simulink library "FG_Controller_Library"  (R2017b)
settings: Solver=VariableStepAuto  StartTime=0.0  StopTime=10.0  RelTol=1e-3
undefined symbols (not defined in the file or in its folder): fcut_velocity_joint, GaitLibrary, isSim, UserParams
libraries: slrtlib x113, simulink x1, func_block_library x1
(part 1 of 3)
settings Model: Creator=81068  LastModifiedBy=hanli

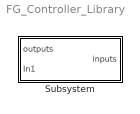
== system FG_Controller_Library ==
  Subsystem : Subsystem

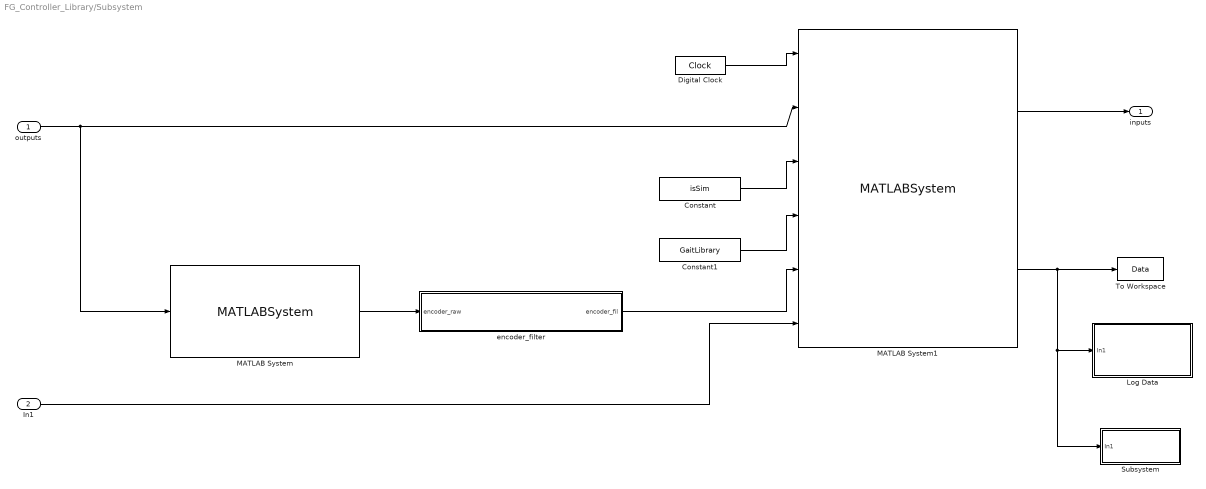
== system FG_Controller_Library/Subsystem ==
  outputs : Inport  OutDataTypeStr=Bus: CassieOutBus
  In1 : Inport  Port=2
  Constant : Constant  Value=isSim  OutDataTypeStr=boolean  LockScale=on
  Constant1 : Constant  Value=GaitLibrary  OutDataTypeStr=Bus: cassieGaitLibraryBus  LockScale=on
  Digital Clock : DigitalClock  SampleTime=UserParams.SampleTime
  Log Data : Subsystem
  MATLAB System : MATLABSystem  System=ExtractJointPosition  SimulateUsing=Code generation
      mask Type: ExtractJointPosition
      mask Display:
      | disp('ExtractJointPosition');
      | port_label('input',1,'cassieOutputs');
      | port_label('output',1,'JointPosition');
  MATLAB System1 : MATLABSystem  System=FG_Controller  Kp_pitch=c_Kp_pitch  Kd_pitch=c_Kd_pitch  Kp_roll=c_Kp_roll  Kd_roll=c_Kd_roll  Kp_yaw=c_Kp_yaw  Kd_yaw=c_Kd_yaw  Kp_abduction=c_Kp_abduction  Kp_rotation=c_Kp_rotation  Kp_thigh=c_Kp_thigh  Kp_knee=c_Kp_knee  Kp_toe=c_Kp_toe  Kd_abduction=c_Kd_abduction  Kd_rotation=c_Kd_rotation  Kd_thigh=c_Kd_thigh  Kd_knee=c_Kd_knee  Kd_toe=c_Kd_toe  Kfs_p=c_Kfs_p  Kfl_p=c_Kfl_p  Kfs_d=c_Kfs_d  Kfl_d=c_Kfl_d  Kp_toe_stand=c_Kp_toe_stand  Kd_toe_stand=c_Kd_toe_stand  Kp_lateral_stand=c_Kp_lateral_stand  Kd_lateral_stand=c_Kd_lateral_stand  Kp_abduction_stand=c_Kp_abduction_stand  Kd_abduction_stand=c_Kd_abduction_stand  Kp_thigh_stand=c_Kp_thigh_stand  Kd_thigh_stand=c_Kd_thigh_stand  Kp_knee_stand=c_Kp_knee_stand  Kd_knee_stand=c_Kd_knee_stand  Kp_rotation_stand=c_Kp_rotation_stand  Kd_rotation_stand=c_Kd_rotation_stand  fil_para_x=c_fil_para_x  fil_para_y=c_fil_para_y  stance_thre_ub=c_stance_thre_ub  stance_thre_lb=c_stance_thre_lb  lateral_velocity_weight=c_lateral_velocity_weight  init_lateral_velocity=c_init_lateral_velocity  abduction_inward_gain=c_abduction_inward_gain  joint_filter_choice=c_joint_filter_choice  shift_time=c_shift_time  shift_distance=c_shift_distance  standing_switch_time=c_standing_switch_time  toe_tilt_angle=c_toe_tilt_angle  final_sw_abduction=c_final_sw_abduction  final_st_abduction=c_final_st_abduction  pre_final_sw_abduction=c_pre_final_sw_abduction  sagittal_offset_exp=c_sagittal_offset_exp  lateral_offset_exp=c_lateral_offset_exp  turning_offset_exp=c_turning_offset_exp  stand_offset_exp=c_stand_offset_exp  u_abduction_cp=c_u_abduction_cp  u_abduction_swing_cp=c_u_abduction_swing_cp  u_thigh_cp=c_u_thigh_cp  u_knee_cp=c_u_knee_cp  fil_para_2=c_fil_para_2  fil_para_3=c_fil_para_3  fil_para_4=c_fil_para_4  fil_para_5=c_fil_para_5  force_step_end_s=c_force_step_end_s  SimulateUsing=Code generation
      mask Type: FG_Controller
      mask Display:
      | disp('FG_Controller');
      | port_label('output',1,'userInputs');
      | port_label('output',2,'Data');
  Subsystem : Subsystem
  To Workspace : ToWorkspace  VariableName=Data  SaveFormat=Timeseries  SampleTime=-1
  encoder_filter : Subsystem  TreatAsAtomicUnit=on
  "inputs " : Outport
  wires:
  outputs/1 -> MATLAB System1/2, MATLAB System/1
  MATLAB System/1 -> encoder_filter/1(encoder_raw)
  encoder_filter/1(encoder_fil) -> MATLAB System1/5
  MATLAB System1/1 -> "inputs "/1
  MATLAB System1/2 -> Subsystem/1(In1), Log Data/1(In1), To Workspace/1
  Digital Clock/1 -> MATLAB System1/1
  Constant/1 -> MATLAB System1/3
  Constant1/1 -> MATLAB System1/4
  In1/1 -> MATLAB System1/6

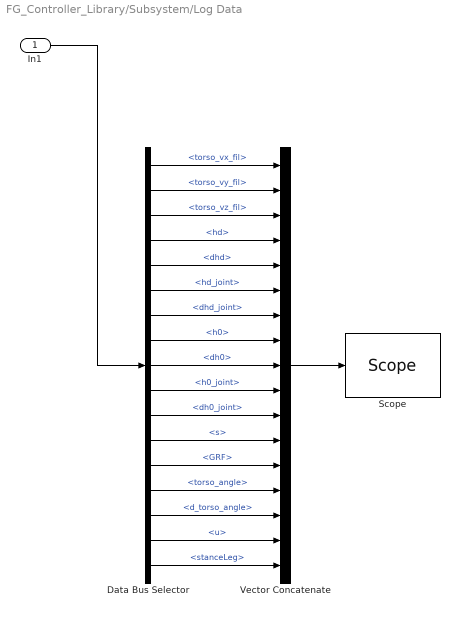
== system FG_Controller_Library/Subsystem/Log Data ==
  In1 : Inport  OutDataTypeStr=Bus: cassieDataBus
  Data Bus Selector : BusSelector  OutputSignals=torso_vx_fil,torso_vy_fil,torso_vz_fil,hd,dhd,hd_joint,dhd_joint,h0,dh0,h0_joint,dh0_joint,s,GRF,torso_angle,d_torso_angle,u,stanceLeg
  "Scope " : slrtlib/Displays and Logging/Scope   scopeno=5  scopetype=File  autostart=on  viewmode=Graphical redraw  formatstr='%15.6f'  grid=on  ylimits=[0,0]  nosamples=250  noprepostsamples=0  interleave=1  triggermode=FreeRun  triggersignal=1  trigsignalfromport=off  triggerlevel=0.0  triggerslope=Either  triggerscope=1  triggersample=0  filename=data.dat  mode=Lazy  writesize=512*8  autorestart=on  dynamicfilemode=off  maxwritefilesize=4*1024^3
  Vector Concatenate : Concatenate  NumInputs=17
  wires:
  In1/1 -> Data Bus Selector/1
  Vector Concatenate/1 -> "Scope "/1
  Data Bus Selector/7 -> Vector Concatenate/7  "<dhd_joint>"
  Data Bus Selector/8 -> Vector Concatenate/8  "<h0>"
  Data Bus Selector/9 -> Vector Concatenate/9  "<dh0>"
  Data Bus Selector/10 -> Vector Concatenate/10  "<h0_joint>"
  Data Bus Selector/3 -> Vector Concatenate/3  "<torso_vz_fil>"
  Data Bus Selector/2 -> Vector Concatenate/2  "<torso_vy_fil>"
  Data Bus Selector/6 -> Vector Concatenate/6  "<hd_joint>"
  Data Bus Selector/1 -> Vector Concatenate/1  "<torso_vx_fil>"
  Data Bus Selector/5 -> Vector Concatenate/5  "<dhd>"
  Data Bus Selector/4 -> Vector Concatenate/4  "<hd>"
  Data Bus Selector/13 -> Vector Concatenate/13  "<GRF>"
  Data Bus Selector/14 -> Vector Concatenate/14  "<torso_angle>"
  Data Bus Selector/15 -> Vector Concatenate/15  "<d_torso_angle>"
  Data Bus Selector/11 -> Vector Concatenate/11  "<dh0_joint>"
  Data Bus Selector/12 -> Vector Concatenate/12  "<s>"
  Data Bus Selector/16 -> Vector Concatenate/16  "<u>"
  Data Bus Selector/17 -> Vector Concatenate/17  "<stanceLeg>"
